simulink model "Symmetry_REAL_TIME"  (Simulink 8.3)
settings: Solver=ode45  StartTime=0.0  StopTime=tfin  RelTol=1e-3
values from neighbouring files (symbols this model uses):
  C = 0    [Sketch_controller_model_ini.m]    (also in Symmetry_REAL_TIME_ini.m = 0.005; Symmetry_ini_Modulary.m = 0.02)
  L = 0    [Sketch_controller_model_ini.m]    (also in Symmetry_REAL_TIME_ini.m = 0.01125)
  Phase_Source = [0,2/3*pi,4/3*pi]    [Sketch_controller_model_ini.m]    (also in Symmetry_REAL_TIME_ini.m; Symmetry_ini.m; Symmetry_ini_COPY.m = [0,-2/3*pi,-4/3*pi])
  R = 100    [Sketch_controller_model_ini.m]    (also in Symmetry_REAL_TIME_ini.m; Symmetry_ini_Modulary.m = 50)
  R_c = 0.005    [Sketch_controller_model_ini.m]    (also in Symmetry_REAL_TIME_ini.m)
  R_l = 0.5    [Sketch_controller_model_ini.m]    (also in Symmetry_REAL_TIME_ini.m)
  sample = 10e-5    (= 0.0001)    [Inverter_ini.m]    (also in Sketch_controller_model_ini.m; Symmetry_REAL_TIME_ini.m; Symmetry_ini.m; Symmetry_ini_COPY.m)
  Urms_Source = [230,230,230]    [Sketch_controller_model_ini.m]    (also in Symmetry_REAL_TIME_ini.m; Symmetry_ini.m; Symmetry_ini_COPY.m)
libraries: powerlib x14, commsequence2 x6, dspxfrm3 x3
settings Model: Creator=Neukirchner László  LastModifiedBy=Templomos
settings DataIOCC: SignalLoggingSaveFormat=Dataset
settings GRTTargetCC: CombineOutputUpdateFcns=on  GRTInterface=off

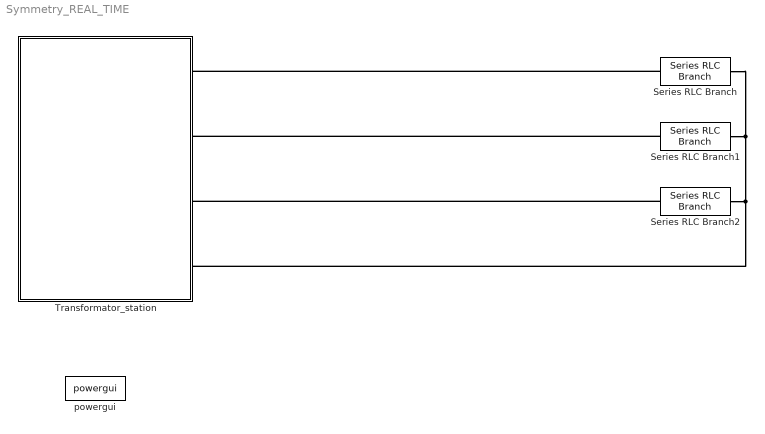
== system Symmetry_REAL_TIME ==
  Series RLC Branch : powerlib/Elements/Series RLC Branch  LConnTagsString=__new0  RConnTagsString=__new0  BranchType=R  Resistance=R  Inductance=L  SetiL0=off  InitialCurrent=0  Capacitance=1e-6  Setx0=off  InitialVoltage=0  Measurements=None
  Series RLC Branch1 : powerlib/Elements/Series RLC Branch  LConnTagsString=__new0  RConnTagsString=__new0  BranchType=RL  Resistance=R_l  Inductance=L  SetiL0=off  InitialCurrent=0  Capacitance=1e-6  Setx0=off  InitialVoltage=0  Measurements=None
  Series RLC Branch2 : powerlib/Elements/Series RLC Branch  LConnTagsString=__new0  RConnTagsString=__new0  BranchType=RC  Resistance=R_c  Inductance=1e-3  SetiL0=off  InitialCurrent=0  Capacitance=C  Setx0=off  InitialVoltage=0  Measurements=None
  Transformator_station : Subsystem
  powergui : powerlib/powergui  SimulationMode=Continuous  SolverType=Tustin  SampleTime=50e-6  frequency=60  SPID=off  DisableSnubberDevices=off  DisableRonSwitches=off  DisableVfSwitches=off  SwTol=0  Interpol=off  DisplayEquations=off  Ts=0  methode=off  frequencyindice=0  Pbase=100e6  ErrMax=1e-4  Iterations=50  UnitsV=kV  UnitsW=MW  FunctionMessages=off  echomessages=off  HookPort=off  EnableUseOfTLC=off  x0status=blocks  RestoreLinks=warning  ResistiveCurrentMeasurement=off  Frange=[0:2:500]  Ylog=off  Xlog=on  ShowGrid=off  save=off  variable=ZData  structure=0  ZoomFFT=on  StartTime=0.0  cycles=1  DisplayStyle=1  fundamental=60  FreqAxis=off  MaxFrequency=1000  frequencyindicesteady=1  RmsSteady=1  display=off
  connections:
  Series RLC Branch/LConn1 -- Transformator_station/RConn1
  Series RLC Branch2/LConn1 -- Transformator_station/RConn3
  Series RLC Branch1/LConn1 -- Transformator_station/RConn2
  Series RLC Branch/RConn1 -- Series RLC Branch1/RConn1 -- Series RLC Branch2/RConn1 -- Transformator_station/RConn4

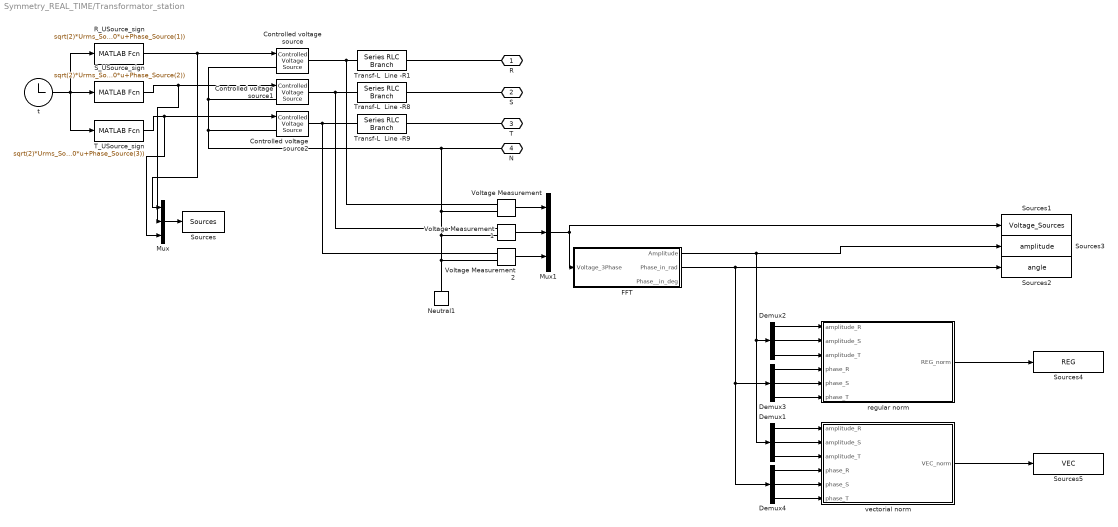
== system Symmetry_REAL_TIME/Transformator_station ==
  " R_USource_sign" : MATLABFcn  MATLABFcn=sqrt(2)*Urms_Source(1)*sin(2*pi*50*u+Phase_Source(1))  SampleTime=sample
  " S_USource_sign" : MATLABFcn  MATLABFcn=sqrt(2)*Urms_Source(2)*sin(2*pi*50*u+Phase_Source(2))  SampleTime=sample
  " T_USource_sign" : MATLABFcn  MATLABFcn=sqrt(2)*Urms_Source(3)*sin(2*pi*50*u+Phase_Source(3))  SampleTime=sample
  Controlled voltage source : powerlib/Electrical Sources/Controlled Voltage Source  Initialize=off  Source_Type=AC  Amplitude=0  Phase=0  Frequency=0  Measurements=None
  Controlled voltage source1 : powerlib/Electrical Sources/Controlled Voltage Source  Initialize=off  Source_Type=AC  Amplitude=0  Phase=0  Frequency=0  Measurements=None
  Controlled voltage source2 : powerlib/Electrical Sources/Controlled Voltage Source  Initialize=off  Source_Type=AC  Amplitude=0  Phase=0  Frequency=0  Measurements=None
  Demux{1..4} (4 alike) : Demux  Outputs=3
  FFT : Subsystem
  Mux : Mux  Inputs=3
  Mux1 : Mux  Inputs=3
  Neutral1 : powerlib/Elements/Neutral  LConnTagsString=a  NodeNumber=10
  Sources : ToWorkspace  VariableName=Sources  SaveFormat=Structure With Time  SampleTime=-1
  Sources1 : ToWorkspace  VariableName=Voltage_Sources  SaveFormat=Structure With Time  SampleTime=sample
  Sources2 : ToWorkspace  VariableName=angle  SaveFormat=Structure With Time  SampleTime=sample
  Sources3 : ToWorkspace  VariableName=amplitude  SaveFormat=Structure With Time  SampleTime=sample
  Sources4 : ToWorkspace  VariableName=REG  SaveFormat=Structure With Time  SampleTime=sample
  Sources5 : ToWorkspace  VariableName=VEC  SaveFormat=Structure With Time  SampleTime=sample
  Transf-L  Line -R1 : powerlib/Elements/Series RLC Branch  LConnTagsString=__new0  RConnTagsString=__new0  BranchType=RL  Resistance=0.4  Inductance=0.003185  SetiL0=off  InitialCurrent=0  Capacitance=1.0  Setx0=off  InitialVoltage=0  Measurements=None
  Transf-L  Line -R8 : powerlib/Elements/Series RLC Branch  LConnTagsString=__new0  RConnTagsString=__new0  BranchType=RL  Resistance=0.4  Inductance=0.003185  SetiL0=off  InitialCurrent=0  Capacitance=1.0  Setx0=off  InitialVoltage=0  Measurements=None
  Transf-L  Line -R9 : powerlib/Elements/Series RLC Branch  LConnTagsString=__new0  RConnTagsString=__new0  BranchType=RL  Resistance=0.4  Inductance=0.003185  SetiL0=off  InitialCurrent=0  Capacitance=1.0  Setx0=off  InitialVoltage=0  Measurements=None
  Voltage Measurement : powerlib/Measurements/Voltage Measurement  PhasorSimulation=off  OutputType=Complex  PSBequivalent=0
  Voltage Measurement1 : powerlib/Measurements/Voltage Measurement  PhasorSimulation=off  OutputType=Complex  PSBequivalent=0
  Voltage Measurement2 : powerlib/Measurements/Voltage Measurement  PhasorSimulation=off  OutputType=Complex  PSBequivalent=0
  regular norm : MATLAB Function  TreatAsAtomicUnit=on
  t : Clock
      settings: Decimation=CLK
  vectorial norm : MATLAB Function  TreatAsAtomicUnit=on
  R : PMIOPort  Port=1  Side=Right
  S : PMIOPort  Port=2  Side=Right
  T : PMIOPort  Port=3  Side=Right
  N : PMIOPort  Port=4  Side=Right
  wires:
  Mux/1 -> Sources/1
  " R_USource_sign"/1 -> Mux/1, Controlled voltage source/1
  " S_USource_sign"/1 -> Mux/2, Controlled voltage source1/1
  " T_USource_sign"/1 -> Mux/3, Controlled voltage source2/1
  t/1 -> " R_USource_sign"/1, " T_USource_sign"/1, " S_USource_sign"/1
  Voltage Measurement/1 -> Mux1/1
  Voltage Measurement2/1 -> Mux1/3
  Mux1/1 -> FFT/1(Voltage_3Phase), Sources1/1
  Voltage Measurement1/1 -> Mux1/2
  regular norm/1(REG_norm) -> Sources4/1
  Demux2/1 -> regular norm/1(amplitude_R)
  Demux2/2 -> regular norm/2(amplitude_S)
  Demux2/3 -> regular norm/3(amplitude_T)
  Demux3/1 -> regular norm/4(phase_R)
  Demux3/2 -> regular norm/5(phase_S)
  Demux3/3 -> regular norm/6(phase_T)
  Demux1/1 -> vectorial norm/1(amplitude_R)
  Demux1/2 -> vectorial norm/2(amplitude_S)
  Demux1/3 -> vectorial norm/3(amplitude_T)
  Demux4/1 -> vectorial norm/4(phase_R)
  Demux4/2 -> vectorial norm/5(phase_S)
  Demux4/3 -> vectorial norm/6(phase_T)
  vectorial norm/1(VEC_norm) -> Sources5/1
  FFT/1(Amplitude) -> Demux1/1, Demux2/1, Sources3/1
  FFT/2(Phase_in_rad) -> Demux4/1, Demux3/1, Sources2/1
  connections:
  Transf-L  Line -R8/RConn1 -- S/RConn1
  Transf-L  Line -R9/RConn1 -- T/RConn1
  Transf-L  Line -R1/RConn1 -- R/RConn1
  Controlled voltage source1/RConn1 -- Voltage Measurement1/LConn1 -- Transf-L  Line -R8/LConn1
  Controlled voltage source2/RConn1 -- Voltage Measurement2/LConn1 -- Transf-L  Line -R9/LConn1
  Transf-L  Line -R1/LConn1 -- Voltage Measurement/LConn1 -- Controlled voltage source/RConn1
  N/RConn1 -- Controlled voltage source/LConn1 -- Controlled voltage source1/LConn1 -- Controlled voltage source2/LConn1 -- Voltage Measurement2/LConn2 -- Neutral1/LConn1 -- Voltage Measurement1/LConn2 -- Voltage Measurement/LConn2

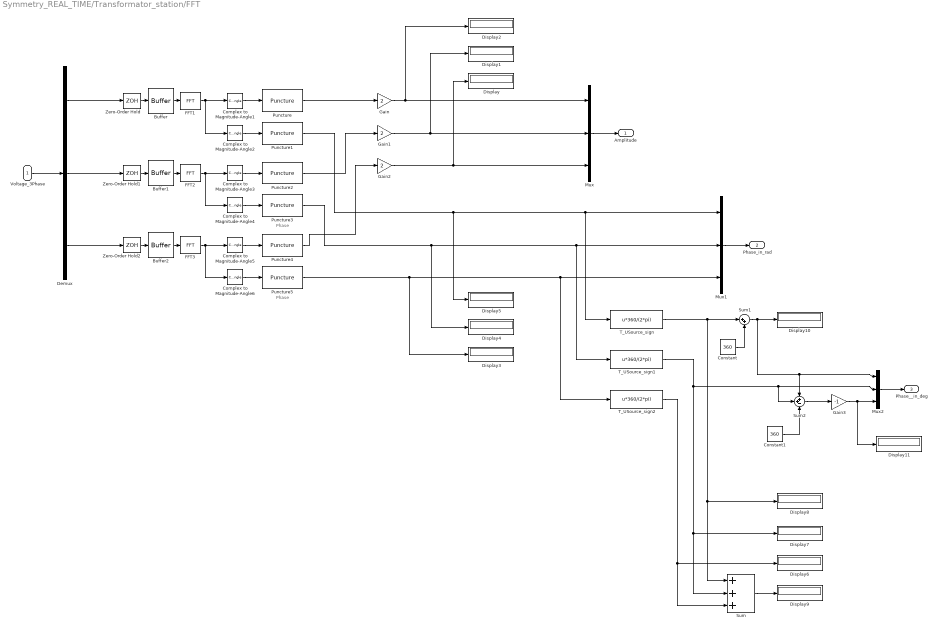
== system Symmetry_REAL_TIME/Transformator_station/FFT ==
  note: Phase
  note: Phase
  Voltage_3Phase : Inport
  " T_USource_sign" : MATLABFcn  MATLABFcn=u*360/(2*pi)  SampleTime=sample
  " T_USource_sign1" : MATLABFcn  MATLABFcn=u*360/(2*pi)  SampleTime=sample
  " T_USource_sign2" : MATLABFcn  MATLABFcn=u*360/(2*pi)  SampleTime=sample
  Buffer : Buffer  N=128
  Buffer1 : Buffer  N=128
  Buffer2 : Buffer  N=128
  Complex to Magnitude-Angle1 : ComplexToMagnitudeAngle  Output=Magnitude
  Complex to Magnitude-Angle2 : ComplexToMagnitudeAngle  Output=Angle
  Complex to Magnitude-Angle3 : ComplexToMagnitudeAngle  Output=Magnitude
  Complex to Magnitude-Angle4 : ComplexToMagnitudeAngle  Output=Angle
  Complex to Magnitude-Angle5 : ComplexToMagnitudeAngle  Output=Magnitude
  Complex to Magnitude-Angle6 : ComplexToMagnitudeAngle  Output=Angle
  Constant : Constant  Value=360
  Constant1 : Constant  Value=360
  Demux : Demux  Outputs=3
  Display{,1..11} (12 alike) : Display
  FFT1 : dspxfrm3/FFT  CompMethod=Table lookup  TableOpt=HYBRID  TableOptActive=Speed  BitRevOrder=off  InheritFFTLength=on  FFTLength=64  WrapInput=on  RowConvenienceOn=on  FFTImplementation=Auto  SkipNorm=on  firstCoeffDataTypeStr=Inherit: Same word length as input  firstCoeffLastDataTypeStr=Inherit: Same word length as input  outputMin=[]  outputMax=[]  roundingMode=Floor  overflowMode=off
  FFT2 : dspxfrm3/FFT  CompMethod=Table lookup  TableOpt=HYBRID  TableOptActive=Speed  BitRevOrder=off  InheritFFTLength=on  FFTLength=64  WrapInput=on  RowConvenienceOn=on  FFTImplementation=Auto  SkipNorm=on  firstCoeffDataTypeStr=Inherit: Same word length as input  firstCoeffLastDataTypeStr=Inherit: Same word length as input  outputMin=[]  outputMax=[]  roundingMode=Floor  overflowMode=off
  FFT3 : dspxfrm3/FFT  CompMethod=Table lookup  TableOpt=HYBRID  TableOptActive=Speed  BitRevOrder=off  InheritFFTLength=on  FFTLength=64  WrapInput=on  RowConvenienceOn=on  FFTImplementation=Auto  SkipNorm=on  firstCoeffDataTypeStr=Inherit: Same word length as input  firstCoeffLastDataTypeStr=Inherit: Same word length as input  outputMin=[]  outputMax=[]  roundingMode=Floor  overflowMode=off
  Gain : Gain  Gain=2  SampleTime=sample
  Gain1 : Gain  Gain=2  SampleTime=sample
  Gain2 : Gain  Gain=2  SampleTime=sample
  Gain3 : Gain  Gain=-1  SampleTime=sample
  Mux : Mux  Inputs=3
  Mux1 : Mux  Inputs=3
  Mux2 : Mux  Inputs=3
  Puncture{,1..5} (6 alike) : commsequence2/Puncture  punctureVector=s'
  Sum : Sum  Inputs=+++
  Sum1 : Sum  Inputs=|++
  Sum2 : Sum  Inputs=++-
  Zero-Order Hold : ZeroOrderHold  SampleTime=20e-3/128
  Zero-Order Hold1 : ZeroOrderHold  SampleTime=20e-3/128
  Zero-Order Hold2 : ZeroOrderHold  SampleTime=20e-3/128
  Amplitude : Outport
  Phase_in_rad : Outport  Port=2
  Phase__in_deg : Outport  Port=3
  wires:
  FFT1/1 -> Complex to Magnitude-Angle1/1, Complex to Magnitude-Angle2/1
  Buffer/1 -> FFT1/1
  Zero-Order Hold/1 -> Buffer/1
  Complex to Magnitude-Angle1/1 -> Puncture/1
  Complex to Magnitude-Angle2/1 -> Puncture1/1
  FFT2/1 -> Complex to Magnitude-Angle4/1, Complex to Magnitude-Angle3/1
  Buffer1/1 -> FFT2/1
  Zero-Order Hold1/1 -> Buffer1/1
  Complex to Magnitude-Angle3/1 -> Puncture2/1
  Complex to Magnitude-Angle4/1 -> Puncture3/1
  FFT3/1 -> Complex to Magnitude-Angle5/1, Complex to Magnitude-Angle6/1
  Buffer2/1 -> FFT3/1
  Zero-Order Hold2/1 -> Buffer2/1
  Complex to Magnitude-Angle5/1 -> Puncture4/1
  Complex to Magnitude-Angle6/1 -> Puncture5/1
  Voltage_3Phase/1 -> Demux/1
  Demux/2 -> Zero-Order Hold1/1
  Demux/3 -> Zero-Order Hold2/1
  Puncture/1 -> Gain/1
  Puncture2/1 -> Gain1/1
  Puncture4/1 -> Gain2/1
  Puncture1/1 -> Display5/1, " T_USource_sign"/1, Mux1/1
  Puncture3/1 -> Display4/1, " T_USource_sign1"/1, Mux1/2
  Puncture5/1 -> Display3/1, " T_USource_sign2"/1, Mux1/3
  Mux/1 -> Amplitude/1
  Mux1/1 -> Phase_in_rad/1
  Gain/1 -> Display2/1, Mux/1
  Gain1/1 -> Display1/1, Mux/2
  Gain2/1 -> Display/1, Mux/3
  Demux/1 -> Zero-Order Hold/1
  " T_USource_sign"/1 -> Sum/1, Display8/1, Sum1/1
  " T_USource_sign1"/1 -> Sum/2, Display7/1, Sum2/2, Mux2/2
  " T_USource_sign2"/1 -> Sum/3, Display6/1
  Sum/1 -> Display9/1
  Constant/1 -> Sum1/2
  Sum1/1 -> Sum2/1, Mux2/1, Display10/1
  Mux2/1 -> Phase__in_deg/1
  Constant1/1 -> Sum2/3
  Gain3/1 -> Display11/1, Mux2/3
  Sum2/1 -> Gain3/1

== matlab function Transformator_station/regular norm ==
  data: amplitude_R input double; REG_norm output double; amplitude_S input double; amplitude_T input double; phase_R input double; phase_S input double; phase_T input double
function REG_norm = fcn(amplitude_R,amplitude_S,amplitude_T,phase_R,phase_S,phase_T)
%#codegen

 A=(1/3)*[1,                1,                  1;...
          1,      exp(1i*120/360*2*pi),        exp(1i*240/360*2*pi);...
          1,      exp(1i*240/360*2*pi),       exp(1i*120/360*2*pi)];
   
   V_real=complex([0,0,0]');
   V_012=complex([0,0,0]');
   V_real(1)=amplitude_R.*exp(1i*phase_R);
   V_real(2)=amplitude_S.*exp(1i*phase_S);
   V_real(3)=amplitude_T.*exp(1i*phase_T); 
   V_012=A*V_real;
   REG_norm=(abs(V_012(3))/abs(V_012(2)))*100;

== matlab function Transformator_station/vectorial norm ==
  data: amplitude_R input double; VEC_norm output double; amplitude_S input double; amplitude_T input double; phase_R input double; phase_S input double; phase_T input double
function VEC_norm = fcn(amplitude_R,amplitude_S,amplitude_T,phase_R,phase_S,phase_T)
%#codegen

   V_real=complex([0,0,0]');
   V_012=complex([0,0,0]');
   N=complex(0);
   V_real(1)=amplitude_R.*exp(1i*phase_R);
   V_real(2)=amplitude_S.*exp(1i*phase_S);
   V_real(3)=amplitude_T.*exp(1i*phase_T);

   R_error=230*exp(1j*0/360*2*pi)  -V_real(1);
   S_error=230*exp(1j*120/360*2*pi)-V_real(2);
   T_error=230*exp(1j*240/360*2*pi)-V_real(3);
   N=R_error*S_error+R_error*T_error+S_error*T_error;
   VEC_norm=abs(N);
